simulink model "Ex3_II"  (R2020b)
settings: Solver=FixedStepAuto  StartTime=0.0  StopTime=10.0  FixedStep=0.001  RelTol=1e-3
settings Model: Creator=macbook  LastModifiedBy=macbook

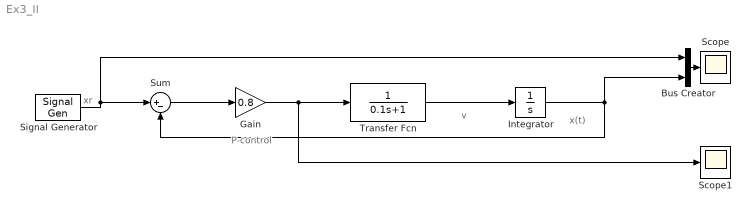
== system Ex3_II ==
  note: xr
  note: x(t)
  note: P-control
  note: v
  Bus Creator : BusCreator  Inputs=2
  Gain : Gain  Gain=0.8
  Integrator : Integrator
  Scope : Scope
  Scope1 : Scope
  Signal Generator : SignalGenerator  Frequency=0.3  Units=rad/sec
  Sum : Sum  Inputs=|+-
  Transfer Fcn : TransferFcn  Numerator=1  Denominator=[0.1 1]
  wires:
  Sum/1 -> Gain/1
  Gain/1 -> Scope1/1, Transfer Fcn/1
  Transfer Fcn/1 -> Integrator/1
  Integrator/1 -> Bus Creator/2, Sum/2
  Signal Generator/1 -> Bus Creator/1, Sum/1
  Bus Creator/1 -> Scope/1
